simulink model "robo_arm_with_control"  (R2018b)
settings: Solver=VariableStepAuto  StartTime=0.0  StopTime=100  RelTol=1e-3  EnableMultiTasking=on
model workspace (MAT data in the model file):
  MCOS : class17 (value not decoded)
undefined symbols (not defined in the file): A_piston, base_rail_height, base_rail_lenth, base_rail_width, border_width_col, box_size_a, D, damp_mech, feedback_loop_gain, first_arm_height, first_arm_length, first_arm_mass, first_arm_width, gearbox_damping_factor, I, jaw_height, jaw_lenght, jaw_mass, jaw_width, K, L_piston, list_of_coordinates_x, list_of_coordinates_y, mechanical_hardstop_constraint, P, pinion_radius, rp_damping_factor, second_arm_height, second_arm_length, second_arm_mass, second_arm_width, third_arm_height, third_arm_length, third_arm_mass, third_arm_width, total_x, winding_resistance, X, x_init, x_max, Y, Z
libraries: fl_lib x47, sm_lib x34, nesl_utility x30, simulink x1, elec_lib x1, SimscapeFluids_lib x1
(part 3 of 3)

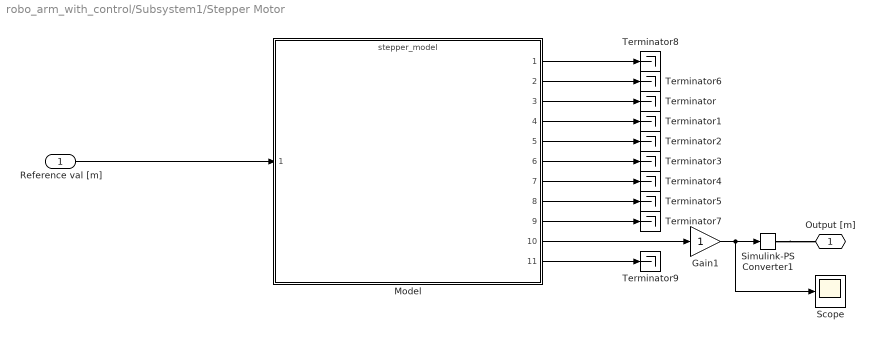
== system robo_arm_with_control/Subsystem1/Stepper Motor  ==
  Reference val [m] : Inport
  Gain1 : Gain
  Model : ModelReference  ModelNameDialog=stepper_model.slx  SimulationMode=Normal  ModelReferenceVersion=1.65
  Scope : Scope
  Simulink-PS Converter1 : nesl_utility/Simulink-PS Converter  PhysicalDomain=network_engine_domain  SubClassName=ps_input  LeftPortType=input  RightPortType=output  PseudoPeriodic=off  Frequencies=[]  NoiseDistribution=none  NoiseParameters=[]  Unit=m  AffineConversion=off  FilteringAndDerivatives=filter  SimscapeFilterOrder=2  InputFilterTimeConstant=0.001  UdotUserProvided=0
  Terminator{,1..9} (10 alike) : Terminator
  Output [m] : PMIOPort  Side=Right
  wires:
  Gain1/1 -> Scope/1, Simulink-PS Converter1/1
  Model/2 -> Terminator6/1
  Model/1 -> Terminator8/1
  Model/3 -> Terminator/1
  Model/4 -> Terminator1/1
  Model/7 -> Terminator4/1
  Model/8 -> Terminator5/1
  Model/9 -> Terminator7/1
  Model/6 -> Terminator3/1
  Model/5 -> Terminator2/1
  Model/11 -> Terminator9/1
  Model/10 -> Gain1/1
  Reference val [m]/1 -> Model/1
  connections:
  Simulink-PS Converter1/RConn1 -- Output [m]/RConn1

== system robo_arm_with_control/Subsystem1/UP//DOWN ==
  Prismatic Joint1 : sm_lib/Joints/Prismatic Joint  SenseConstraintForce=off  SenseConstraintForceX=off  SenseConstraintForceY=off  SenseConstraintForceZ=off  SenseConstraintTorque=off  SenseConstraintTorqueX=off  SenseConstraintTorqueY=off  SenseConstraintTorqueZ=off  SenseTotalForce=off  SenseTotalForceX=off  SenseTotalForceY=off  SenseTotalForceZ=off  SenseTotalTorque=off  SenseTotalTorqueX=off  SenseTotalTorqueY=off  SenseTotalTorqueZ=off  CompositeWrenchDir=FollowerOnBase  CompositeWrenchFrame=BaseFrame  EquilibriumPosition=0  EquilibriumPositionUnits=cm  SpringStiffness=0  SpringStiffnessUnits=N/m  DampingCoefficient=0  DampingCoefficientUnits=N/(m/s)  TorqueActuationMode=ComputedTorque  MotionActuationMode=InputMotion  SensePosition=on  SenseVelocity=off  SenseAcceleration=off  SenseTorqueForce=off  PositionTargetSpecify=off  PositionTargetPriority=High  PositionTargetValue=0  PositionTargetValueUnits=m  VelocityTargetSpecify=off  VelocityTargetPriority=High  VelocityTargetValue=0  VelocityTargetValueUnits=m/s
  In : PMIOPort  Side=Right
  Out : PMIOPort  Port=2  Side=Right
  Ang. Pos. In : PMIOPort  Port=3  Side=Right
  Pos_Out : PMIOPort  Port=4  Side=Right
  connections:
  Prismatic Joint1/LConn1 -- In/RConn1
  Prismatic Joint1/RConn1 -- Out/RConn1
  Ang. Pos. In/RConn1 -- Prismatic Joint1/LConn2
  Pos_Out/RConn1 -- Prismatic Joint1/RConn2

== system robo_arm_with_control/Subsystem1/X Servo ==
  Prismatic Joint : sm_lib/Joints/Prismatic Joint  SenseConstraintForce=off  SenseConstraintForceX=off  SenseConstraintForceY=off  SenseConstraintForceZ=off  SenseConstraintTorque=off  SenseConstraintTorqueX=off  SenseConstraintTorqueY=off  SenseConstraintTorqueZ=off  SenseTotalForce=off  SenseTotalForceX=off  SenseTotalForceY=off  SenseTotalForceZ=off  SenseTotalTorque=off  SenseTotalTorqueX=off  SenseTotalTorqueY=off  SenseTotalTorqueZ=off  CompositeWrenchDir=FollowerOnBase  CompositeWrenchFrame=BaseFrame  EquilibriumPosition=0  EquilibriumPositionUnits=cm  SpringStiffness=x_stiffness  SpringStiffnessUnits=N/m  DampingCoefficient=x_damping  DampingCoefficientUnits=N/(m/s)  TorqueActuationMode=ComputedTorque  MotionActuationMode=InputMotion  SensePosition=on  SenseVelocity=off  SenseAcceleration=off  SenseTorqueForce=off  PositionTargetSpecify=off  PositionTargetPriority=High  PositionTargetValue=0  PositionTargetValueUnits=m  VelocityTargetSpecify=off  VelocityTargetPriority=High  VelocityTargetValue=0  VelocityTargetValueUnits=m/s
  Rigid Transform : sm_lib/Frames and Transforms/Rigid Transform  TranslationMethod=None  TranslationStandardOffset=0  TranslationLengthUnit=m  TranslationStandardAxis=+Z  TranslationCartesianOffset=[0 0 0]  TranslationROffset=0  TranslationROffsetUnits=m  TranslationZOffset=0  TranslationZOffsetUnits=m  TranslationThetaOffset=0  TranslationThetaOffsetUnits=deg  RotationMethod=StandardAxis  RotationAngleUnits=deg  RotationStandardAxis=+Y  RotationAngle=90  RotationArbitraryAxis=[0 0 1]  FollAlignAxisA=+X  BaseAlignAxisA=+Y  FollAlignAxisB=+Y  BaseAlignAxisB=+Z  RotationSequenceAxes=FollowerAxes  RotationSequence=XYX  RotationSequenceAngles=[0 0 0]  RotationSequenceAnglesUnits=deg  RotationMatrix=[1 0 0; 0 1 0; 0 0 1]
  Rigid Transform1 : sm_lib/Frames and Transforms/Rigid Transform  TranslationMethod=None  TranslationStandardOffset=0  TranslationLengthUnit=m  TranslationStandardAxis=+Z  TranslationCartesianOffset=[0 0 0]  TranslationROffset=0  TranslationROffsetUnits=m  TranslationZOffset=0  TranslationZOffsetUnits=m  TranslationThetaOffset=0  TranslationThetaOffsetUnits=deg  RotationMethod=StandardAxis  RotationAngleUnits=deg  RotationStandardAxis=+Y  RotationAngle=90  RotationArbitraryAxis=[0 0 1]  FollAlignAxisA=+X  BaseAlignAxisA=+Y  FollAlignAxisB=+Y  BaseAlignAxisB=+Z  RotationSequenceAxes=FollowerAxes  RotationSequence=XYX  RotationSequenceAngles=[0 0 0]  RotationSequenceAnglesUnits=deg  RotationMatrix=[1 0 0; 0 1 0; 0 0 1]
  In : PMIOPort  Side=Right
  Out : PMIOPort  Port=2  Side=Right
  Ang. Pos. Input : PMIOPort  Port=3  Side=Left
  Pos_Out : PMIOPort  Port=4  Side=Right
  connections:
  In/RConn1 -- Rigid Transform1/RConn1
  Prismatic Joint/LConn1 -- Rigid Transform1/LConn1
  Out/RConn1 -- Rigid Transform/RConn1
  Prismatic Joint/RConn1 -- Rigid Transform/LConn1
  Ang. Pos. Input/RConn1 -- Prismatic Joint/LConn2
  Pos_Out/RConn1 -- Prismatic Joint/RConn2

== system robo_arm_with_control/Subsystem1/Y Servo ==
  Prismatic Joint1 : sm_lib/Joints/Prismatic Joint  SenseConstraintForce=off  SenseConstraintForceX=off  SenseConstraintForceY=off  SenseConstraintForceZ=off  SenseConstraintTorque=off  SenseConstraintTorqueX=off  SenseConstraintTorqueY=off  SenseConstraintTorqueZ=off  SenseTotalForce=off  SenseTotalForceX=off  SenseTotalForceY=off  SenseTotalForceZ=off  SenseTotalTorque=off  SenseTotalTorqueX=off  SenseTotalTorqueY=off  SenseTotalTorqueZ=off  CompositeWrenchDir=FollowerOnBase  CompositeWrenchFrame=BaseFrame  EquilibriumPosition=0  EquilibriumPositionUnits=cm  SpringStiffness=0  SpringStiffnessUnits=N/m  DampingCoefficient=0  DampingCoefficientUnits=N/(m/s)  TorqueActuationMode=ComputedTorque  MotionActuationMode=InputMotion  SensePosition=on  SenseVelocity=off  SenseAcceleration=off  SenseTorqueForce=off  PositionTargetSpecify=off  PositionTargetPriority=High  PositionTargetValue=0  PositionTargetValueUnits=m  VelocityTargetSpecify=off  VelocityTargetPriority=High  VelocityTargetValue=0  VelocityTargetValueUnits=m/s
  Rigid Transform3 : sm_lib/Frames and Transforms/Rigid Transform  TranslationMethod=None  TranslationStandardOffset=0  TranslationLengthUnit=m  TranslationStandardAxis=+Z  TranslationCartesianOffset=[0 0 0]  TranslationROffset=0  TranslationROffsetUnits=m  TranslationZOffset=0  TranslationZOffsetUnits=m  TranslationThetaOffset=0  TranslationThetaOffsetUnits=deg  RotationMethod=StandardAxis  RotationAngleUnits=deg  RotationStandardAxis=-X  RotationAngle=90  RotationArbitraryAxis=[0 0 1]  FollAlignAxisA=+X  BaseAlignAxisA=+Y  FollAlignAxisB=+Y  BaseAlignAxisB=+Z  RotationSequenceAxes=FollowerAxes  RotationSequence=XYX  RotationSequenceAngles=[0 0 0]  RotationSequenceAnglesUnits=deg  RotationMatrix=[1 0 0; 0 1 0; 0 0 1]
  Rigid Transform4 : sm_lib/Frames and Transforms/Rigid Transform  TranslationMethod=None  TranslationStandardOffset=0  TranslationLengthUnit=m  TranslationStandardAxis=+Z  TranslationCartesianOffset=[0 0 0]  TranslationROffset=0  TranslationROffsetUnits=m  TranslationZOffset=0  TranslationZOffsetUnits=m  TranslationThetaOffset=0  TranslationThetaOffsetUnits=deg  RotationMethod=StandardAxis  RotationAngleUnits=deg  RotationStandardAxis=-X  RotationAngle=90  RotationArbitraryAxis=[0 0 1]  FollAlignAxisA=+X  BaseAlignAxisA=+Y  FollAlignAxisB=+Y  BaseAlignAxisB=+Z  RotationSequenceAxes=FollowerAxes  RotationSequence=XYX  RotationSequenceAngles=[0 0 0]  RotationSequenceAnglesUnits=deg  RotationMatrix=[1 0 0; 0 1 0; 0 0 1]
  In : PMIOPort  Side=Right
  Out : PMIOPort  Port=2  Side=Right
  Ang. Pos. In : PMIOPort  Port=3  Side=Right
  Pos_Out : PMIOPort  Port=4  Side=Right
  connections:
  In/RConn1 -- Rigid Transform4/RConn1
  Prismatic Joint1/RConn1 -- Rigid Transform3/LConn1
  Prismatic Joint1/LConn1 -- Rigid Transform4/LConn1
  Out/RConn1 -- Rigid Transform3/RConn1
  Ang. Pos. In/RConn1 -- Prismatic Joint1/LConn2
  Prismatic Joint1/RConn2 -- Pos_Out/RConn1

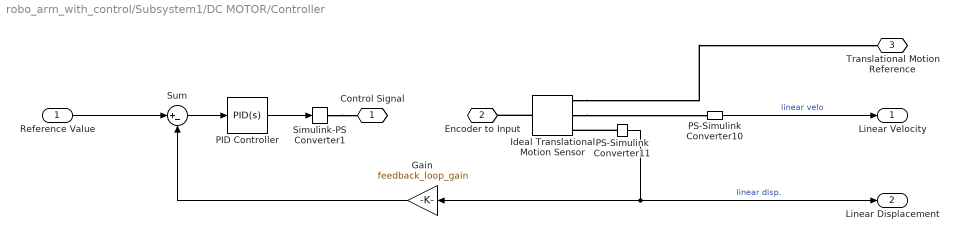
== system robo_arm_with_control/Subsystem1/DC MOTOR/Controller ==
  Reference Value : Inport
  Gain : Gain  Gain=feedback_loop_gain
  Ideal Translational Motion Sensor : fl_lib/Mechanical/Mechanical Sensors/Ideal Translational Motion Sensor  offset=0 m
  PID Controller : simulink/Continuous/PID Controller  Controller=PID  Form=Parallel  TimeDomain=Continuous-time  SampleTime=-1  IntegratorMethod=Forward Euler  FilterMethod=Forward Euler  ControllerParametersSource=internal  P=P  I=I  D=D  UseFilter=on  N=100  TunerSelectOption=Transfer Function Based (PID Tuner App)  InitialConditionSource=internal  InitialConditionForIntegrator=0  InitialConditionForFilter=0  DifferentiatorICPrevScaledInput=0  ExternalReset=none  TrackingMode=off  Kt=1  LimitOutput=off  UpperSaturationLimit=inf  LowerSaturationLimit=-inf  LinearizeAsGain=on  AntiWindupMode=none  Kb=1  POutMin=[]  POutMax=[]  IOutMin=[]  IOutMax=[]  DOutMin=[]  DOutMax=[]  NOutMin=[]  NOutMax=[]  SumOutMin=[]  SumOutMax=[]  SaturationOutMin=[]  SaturationOutMax=[]  PParamMin=[]  PParamMax=[]  IParamMin=[]  IParamMax=[]  DParamMin=[]  DParamMax=[]  NParamMin=[]  NParamMax=[]  KbParamMin=[]  KbParamMax=[]  KtParamMin=[]  KtParamMax=[]  KbOutMin=[]  KbOutMax=[]  KtOutMin=[]  KtOutMax=[]  IntegratorOutMin=[]  IntegratorOutMax=[]  FilterOutMin=[]  FilterOutMax=[]  SumI1OutMin=[]  SumI1OutMax=[]  SumI2OutMin=[]  SumI2OutMax=[]  SumI3OutMin=[]  SumI3OutMax=[]  SumI4OutMin=[]  SumI4OutMax=[]  SumDOutMin=[]  SumDOutMax=[]  DifferentiatorOutMin=[]  DifferentiatorOutMax=[]  FilterDiffOutCoefMin=[]  FilterDiffOutCoefMax=[]  ReciprocalOutMin=[]  ReciprocalOutMax=[]  SumDenOutMin=[]  SumDenOutMax=[]  SumNumOutMin=[]  SumNumOutMax=[]  DivideOutMin=[]  DivideOutMax=[]  IntegratorContinuousStateAttributes=''  IntegratorStateMustResolveToSignalObject=off  IntegratorRTWStateStorageClass=Auto  FilterContinuousStateAttributes=''  FilterStateMustResolveToSignalObject=off  FilterRTWStateStorageClass=Auto  ParallelPVariant=InternalParameters  IdealPVariant=Disabled  IVariant=InternalParameters  DVariant=InternalParameters  IntegratorVariant=Continuous  SatVariant=Disabled  AWVariant=Passthrough  PCopyVariant=Disabled  TRVariant=Disabled  FdbkBlocksVariant=Forward  IdealPFdbkVariant=Disabled  SatFdbkVariant=Disabled  DerivativeFilterVariant=ContFilter  NVariant=InternalParameters  NCopyVariant=Disabled  FilterICVariant=InternalICsFilter  IntegratorICVariant=InternalICs  ExternalResetVariant=Disabled  TRSumVariant=Passthrough  SumFdbkVariant=Disabled  SumVariant=Sum_PID
  PS-Simulink Converter10 : nesl_utility/PS-Simulink Converter  PhysicalDomain=network_engine_domain  SubClassName=ps_output  LeftPortType=input  RightPortType=output  PseudoPeriodic=off  Frequencies=[]  Unit=1  AffineConversion=off
  PS-Simulink Converter11 : nesl_utility/PS-Simulink Converter  PhysicalDomain=network_engine_domain  SubClassName=ps_output  LeftPortType=input  RightPortType=output  PseudoPeriodic=off  Frequencies=[]  Unit=m  AffineConversion=off
  Simulink-PS Converter1 : nesl_utility/Simulink-PS Converter  PhysicalDomain=network_engine_domain  SubClassName=ps_input  LeftPortType=input  RightPortType=output  PseudoPeriodic=off  Frequencies=[]  NoiseDistribution=none  NoiseParameters=[]  Unit=1  AffineConversion=off  FilteringAndDerivatives=filter  SimscapeFilterOrder=1  InputFilterTimeConstant=0.001  UdotUserProvided=0
  Sum : Sum  Inputs=|+-
  Control Signal : PMIOPort  Side=Right
  Encoder to Input : PMIOPort  Port=2  Side=Left
  Translational Motion Reference : PMIOPort  Port=3  Side=Left
  Linear Velocity : Outport
  Linear Displacement : Outport  Port=2
  wires:
  Reference Value/1 -> Sum/1
  PS-Simulink Converter11/1 -> Linear Displacement/1, Gain/1  "linear disp."
  PID Controller/1 -> Simulink-PS Converter1/1
  Sum/1 -> PID Controller/1
  Gain/1 -> Sum/2
  PS-Simulink Converter10/1 -> Linear Velocity/1  "linear velo"
  connections:
  Ideal Translational Motion Sensor/RConn1 -- Translational Motion Reference/RConn1
  Simulink-PS Converter1/RConn1 -- Control Signal/RConn1
  PS-Simulink Converter11/LConn1 -- Ideal Translational Motion Sensor/RConn3
  Ideal Translational Motion Sensor/LConn1 -- Encoder to Input/RConn1
  Ideal Translational Motion Sensor/RConn2 -- PS-Simulink Converter10/LConn1

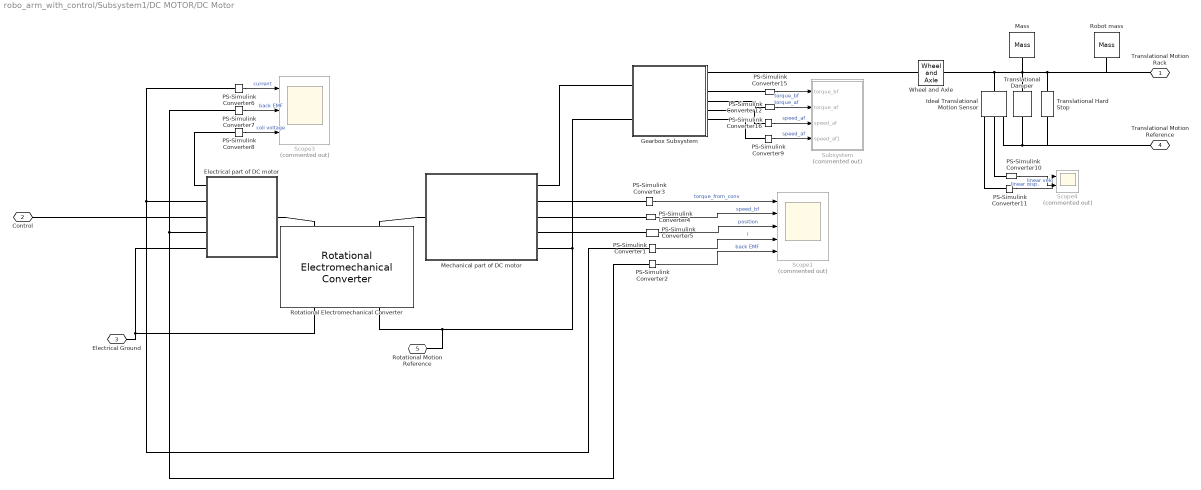
== system robo_arm_with_control/Subsystem1/DC MOTOR/DC Motor ==
  Electrical part of DC motor : Subsystem
  Gearbox Subsystem : Subsystem
  Ideal Translational Motion Sensor : fl_lib/Mechanical/Mechanical Sensors/Ideal Translational Motion Sensor  offset=0 m
  Mass : fl_lib/Mechanical/Translational Elements/Mass  mass=rack_mass kg  v_specify=off  v_priority=High  v=0 m/s  v_nominal_specify=off  v_nominal_unit=m/s  v_nominal_value=1  f_specify=off  f_priority=None  f=0 N  f_nominal_specify=off  f_nominal_unit=N  f_nominal_value=1
  Mechanical part of DC motor : Subsystem
  PS-Simulink Converter{1..12,15..16} (14 alike) : nesl_utility/PS-Simulink Converter  PhysicalDomain=network_engine_domain  SubClassName=ps_output  LeftPortType=input  RightPortType=output  PseudoPeriodic=off  Frequencies=[]  Unit=1  AffineConversion=off
  Robot mass : fl_lib/Mechanical/Translational Elements/Mass  mass=first_arm_mass + second_arm_mass + third_arm_mass + jaw_mass*2 kg  v_specify=off  v_priority=High  v=0 m/s  v_nominal_specify=off  v_nominal_unit=m/s  v_nominal_value=1  f_specify=off  f_priority=None  f=0 N  f_nominal_specify=off  f_nominal_unit=N  f_nominal_value=1
  Rotational Electromechanical Converter : fl_lib/Electrical/Electrical Elements/Rotational Electromechanical Converter  K=K V/rpm  i_specify=off  i_priority=None  i=0 A  i_nominal_specify=off  i_nominal_unit=A  i_nominal_value=1  v_specify=off  v_priority=None  v=0 V  v_nominal_specify=off  v_nominal_unit=V  v_nominal_value=1  t_specify=off  t_priority=None  t=0 N*m  t_nominal_specify=off  t_nominal_unit=N*m  t_nominal_value=1  w_specify=off  w_priority=None  w=0 rad/s  w_nominal_specify=off  w_nominal_unit=rad/s  w_nominal_value=1
      settings: SourceProductName=Simscape
  Scope1 : Scope  Commented=on  NumInputPorts=5
  Scope3 : Scope  Commented=on  NumInputPorts=3
  Scope4 : Scope  Commented=on  NumInputPorts=2
  Subsystem : Subsystem  Commented=on
  Translational Damper : fl_lib/Mechanical/Translational Elements/Translational Damper  D=rp_damping_factor N/(m/s)  v_specify=off  v_priority=None  v=0 m/s  v_nominal_specify=off  v_nominal_unit=m/s  v_nominal_value=1  f_specify=off  f_priority=None  f=0 N  f_nominal_specify=off  f_nominal_unit=N  f_nominal_value=1
  Translational Hard Stop : fl_lib/Mechanical/Translational Elements/Translational Hard Stop  upper_bnd=mechanical_hardstop_constraint m  lower_bnd=-mechanical_hardstop_constraint m  stiff_up=1e6 N/m  stiff_low=1e6 N/m  D_up=150 N/(m/s)  D_low=150 N/(m/s)  model=1  transition=0.1 mm  v_specify=off  v_priority=None  v=0 m/s  v_nominal_specify=off  v_nominal_unit=m/s  v_nominal_value=1  f_specify=off  f_priority=None  f=0 N  f_nominal_specify=off  f_nominal_unit=N  f_nominal_value=1  x_specify=off  x_priority=High  x=0 m  x_nominal_specify=off  x_nominal_unit=m  x_nominal_value=1
  Wheel and Axle : fl_lib/Mechanical/Mechanisms/Wheel and Axle  R=pinion_radius m  or=1  t_specify=off  t_priority=None  t=0 N*m  t_nominal_specify=off  t_nominal_unit=N*m  t_nominal_value=1  f_specify=off  f_priority=None  f=0 N  f_nominal_specify=off  f_nominal_unit=N  f_nominal_value=1
      settings: SourceProductName=Simscape
  Translational Motion Rack : PMIOPort  Side=Right
  Control : PMIOPort  Port=2  Side=Left
  Electrical Ground : PMIOPort  Port=3  Side=Left
  Translational Motion Reference : PMIOPort  Port=4  Side=Left
  Rotational Motion Reference : PMIOPort  Port=5  Side=Left
  wires:
  PS-Simulink Converter1/1 -> Scope1/4  "i"
  PS-Simulink Converter8/1 -> Scope3/3  "coil voltage"
  PS-Simulink Converter15/1 -> Subsystem/1(torque_bf)  "torque_bf"
  PS-Simulink Converter5/1 -> Scope1/3  "position"
  PS-Simulink Converter6/1 -> Scope3/1  "current"
  PS-Simulink Converter9/1 -> Subsystem/4(speed_af1)  "speed_af"
  PS-Simulink Converter7/1 -> Scope3/2  "back EMF"
  PS-Simulink Converter3/1 -> Scope1/1  "torque_from_conv"
  PS-Simulink Converter2/1 -> Scope1/5  "back EMF"
  PS-Simulink Converter11/1 -> Scope4/1  "linear disp."
  PS-Simulink Converter16/1 -> Subsystem/3(speed_af)  "speed_af"
  PS-Simulink Converter10/1 -> Scope4/2  "linear velo"
  PS-Simulink Converter12/1 -> Subsystem/2(torque_af)  "torque_af"
  PS-Simulink Converter4/1 -> Scope1/2  "speed_bf"
  connections:
  Gearbox Subsystem/RConn4 -- PS-Simulink Converter12/LConn1
  Rotational Electromechanical Converter/RConn1 -- Electrical part of DC motor/RConn5 -- Electrical Ground/RConn1
  PS-Simulink Converter4/LConn1 -- Mechanical part of DC motor/RConn3
  PS-Simulink Converter9/LConn1 -- Gearbox Subsystem/RConn6
  Ideal Translational Motion Sensor/RConn3 -- PS-Simulink Converter11/LConn1
  Control/RConn1 -- Electrical part of DC motor/RConn3
  PS-Simulink Converter5/LConn1 -- Mechanical part of DC motor/RConn4
  PS-Simulink Converter16/LConn1 -- Gearbox Subsystem/RConn5
  PS-Simulink Converter6/LConn1 -- PS-Simulink Converter1/LConn1 -- Electrical part of DC motor/RConn2
  Ideal Translational Motion Sensor/LConn1 -- Translational Motion Rack/RConn1 -- Robot mass/LConn1 -- Translational Hard Stop/LConn1 -- Mass/LConn1 -- Translational Damper/LConn1 -- Wheel and Axle/RConn1
  Electrical part of DC motor/LConn1 -- Rotational Electromechanical Converter/LConn1
  PS-Simulink Converter7/LConn1 -- Electrical part of DC motor/RConn4 -- PS-Simulink Converter2/LConn1
  Mechanical part of DC motor/LConn1 -- Rotational Electromechanical Converter/LConn2
  Gearbox Subsystem/LConn1 -- Mechanical part of DC motor/RConn1
  PS-Simulink Converter15/LConn1 -- Gearbox Subsystem/RConn3
  Translational Damper/RConn1 -- Translational Motion Reference/RConn1 -- Translational Hard Stop/RConn1 -- Ideal Translational Motion Sensor/RConn1
  Gearbox Subsystem/LConn2 -- Mechanical part of DC motor/RConn5 -- Rotational Motion Reference/RConn1 -- Rotational Electromechanical Converter/RConn2
  Ideal Translational Motion Sensor/RConn2 -- PS-Simulink Converter10/LConn1
  Mechanical part of DC motor/RConn2 -- PS-Simulink Converter3/LConn1
  Wheel and Axle/LConn1 -- Gearbox Subsystem/RConn1
  Electrical part of DC motor/RConn1 -- PS-Simulink Converter8/LConn1

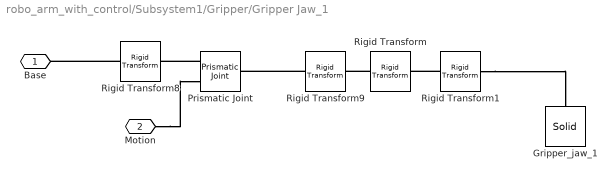
== system robo_arm_with_control/Subsystem1/Gripper/Gripper Jaw_1 ==
  Gripper_jaw_1 : sm_lib/Body Elements/Solid  InertiaType=CalculateFromGeometry  Mass=1  MassUnits=kg  CenterOfMass=[0 0 0]  CenterOfMassUnits=m  MomentsOfInertia=[1 1 1]  MomentsOfInertiaUnits=kg*m^2  ProductsOfInertia=[0 0 0]  ProductsOfInertiaUnits=kg*m^2  BasedOnType=Density  Density=jaw_density  DensityUnits=kg/m^3  DoExposeReferenceFrame=on  SerializedFrames=<Frames/>  GraphicType=FromGeometry  MarkerShape=Sphere  MarkerSize=10  GraphicVisPropType=SimpleVisualProperties  GraphicDiffuseColor=[0.5 0.5 0.5]  GraphicSpecularColor=[0.5 0.5 0.5 1.0]  GraphicAmbientColor=[0.15 0.15 0.15 1.0]  GraphicEmissiveColor=[0.0 0.0 0.0 1.0]  GraphicShininess=75  GraphicOpacity=1.0  GeometryShape=Brick  RectangleSize=[1 1]  RectangleSizeUnits=m  BrickDimensions=[jaw_width jaw_lenght jaw_height]  BrickDimensionUnits=cm  CylinderRadius=1  CylinderRadiusUnits=m  CylinderLength=1  CylinderLengthUnits=m  SphereRadius=1  SphereRadiusUnits=m  EllipsoidRadii=[1 1 1]  EllipsoidRadiiUnits=m  ExtrusionCrossSection=[1 1; -1 1; -1 -1; 1 -1]  ExtrusionCrossSectionUnits=m  ExtrusionLength=1  ExtrusionLengthUnits=m  PolygonNumSides=3  PolygonOuterRadius=1  PolygonOuterRadiusUnits=m  ExtGeomFileType=STEP  ExtGeomFileUnits=m  RevolutionCrossSection=[1 1; 1 -1; 2 -1; 2 1]  RevolutionCrossSectionUnits=m  RevolutionExtent=Full  RevolutionAngle=180  RevolutionAngleUnits=deg
  Prismatic Joint : sm_lib/Joints/Prismatic Joint  SenseConstraintForce=off  SenseConstraintForceX=off  SenseConstraintForceY=off  SenseConstraintForceZ=off  SenseConstraintTorque=off  SenseConstraintTorqueX=off  SenseConstraintTorqueY=off  SenseConstraintTorqueZ=off  SenseTotalForce=off  SenseTotalForceX=off  SenseTotalForceY=off  SenseTotalForceZ=off  SenseTotalTorque=off  SenseTotalTorqueX=off  SenseTotalTorqueY=off  SenseTotalTorqueZ=off  CompositeWrenchDir=FollowerOnBase  CompositeWrenchFrame=BaseFrame  EquilibriumPosition=0  EquilibriumPositionUnits=m  SpringStiffness=0  SpringStiffnessUnits=N/m  DampingCoefficient=0  DampingCoefficientUnits=N/(m/s)  TorqueActuationMode=ComputedTorque  MotionActuationMode=InputMotion  SensePosition=off  SenseVelocity=off  SenseAcceleration=off  SenseTorqueForce=off  PositionTargetSpecify=off  PositionTargetPriority=High  PositionTargetValue=0  PositionTargetValueUnits=m  VelocityTargetSpecify=off  VelocityTargetPriority=High  VelocityTargetValue=0  VelocityTargetValueUnits=m/s
  Rigid Transform : sm_lib/Frames and Transforms/Rigid Transform  TranslationMethod=StandardAxis  TranslationStandardOffset=third_arm_height/2+jaw_height/2  TranslationLengthUnit=cm  TranslationStandardAxis=+Z  TranslationCartesianOffset=[0 0 0]  TranslationROffset=0  TranslationROffsetUnits=m  TranslationZOffset=0  TranslationZOffsetUnits=m  TranslationThetaOffset=0  TranslationThetaOffsetUnits=deg  RotationMethod=None  RotationAngleUnits=deg  RotationStandardAxis=-Z  RotationAngle=0.0  RotationArbitraryAxis=[0 0 1]  FollAlignAxisA=+X  BaseAlignAxisA=+Y  FollAlignAxisB=+Y  BaseAlignAxisB=+Z  RotationSequenceAxes=FollowerAxes  RotationSequence=XYX  RotationSequenceAngles=[0 0 0]  RotationSequenceAnglesUnits=deg  RotationMatrix=[1 0 0; 0 1 0; 0 0 1]
  Rigid Transform1 : sm_lib/Frames and Transforms/Rigid Transform  TranslationMethod=StandardAxis  TranslationStandardOffset=third_arm_length/2+jaw_width/2  TranslationLengthUnit=cm  TranslationStandardAxis=+X  TranslationCartesianOffset=[0 0 0]  TranslationROffset=0  TranslationROffsetUnits=m  TranslationZOffset=0  TranslationZOffsetUnits=m  TranslationThetaOffset=0  TranslationThetaOffsetUnits=deg  RotationMethod=None  RotationAngleUnits=deg  RotationStandardAxis=+Z  RotationAngle=0.0  RotationArbitraryAxis=[0 0 1]  FollAlignAxisA=+X  BaseAlignAxisA=+Y  FollAlignAxisB=+Y  BaseAlignAxisB=+Z  RotationSequenceAxes=FollowerAxes  RotationSequence=XYX  RotationSequenceAngles=[0 0 0]  RotationSequenceAnglesUnits=deg  RotationMatrix=[1 0 0; 0 1 0; 0 0 1]
  Rigid Transform8 : sm_lib/Frames and Transforms/Rigid Transform  TranslationMethod=None  TranslationStandardOffset=0  TranslationLengthUnit=m  TranslationStandardAxis=+Z  TranslationCartesianOffset=[0 0 0]  TranslationROffset=0  TranslationROffsetUnits=m  TranslationZOffset=0  TranslationZOffsetUnits=m  TranslationThetaOffset=0  TranslationThetaOffsetUnits=deg  RotationMethod=StandardAxis  RotationAngleUnits=deg  RotationStandardAxis=+Y  RotationAngle=90  RotationArbitraryAxis=[0 0 1]  FollAlignAxisA=+X  BaseAlignAxisA=+Y  FollAlignAxisB=+Y  BaseAlignAxisB=+Z  RotationSequenceAxes=FollowerAxes  RotationSequence=XYX  RotationSequenceAngles=[0 0 0]  RotationSequenceAnglesUnits=deg  RotationMatrix=[1 0 0; 0 1 0; 0 0 1]
  Rigid Transform9 : sm_lib/Frames and Transforms/Rigid Transform  TranslationMethod=None  TranslationStandardOffset=0  TranslationLengthUnit=m  TranslationStandardAxis=+Z  TranslationCartesianOffset=[0 0 0]  TranslationROffset=0  TranslationROffsetUnits=m  TranslationZOffset=0  TranslationZOffsetUnits=m  TranslationThetaOffset=0  TranslationThetaOffsetUnits=deg  RotationMethod=StandardAxis  RotationAngleUnits=deg  RotationStandardAxis=+Y  RotationAngle=90  RotationArbitraryAxis=[0 0 1]  FollAlignAxisA=+X  BaseAlignAxisA=+Y  FollAlignAxisB=+Y  BaseAlignAxisB=+Z  RotationSequenceAxes=FollowerAxes  RotationSequence=XYX  RotationSequenceAngles=[0 0 0]  RotationSequenceAnglesUnits=deg  RotationMatrix=[1 0 0; 0 1 0; 0 0 1]
  Base : PMIOPort  Side=Left
  Motion : PMIOPort  Port=2  Side=Left
  connections:
  Rigid Transform/LConn1 -- Rigid Transform9/LConn1
  Rigid Transform1/LConn1 -- Rigid Transform/RConn1
  Rigid Transform8/LConn1 -- Base/RConn1
  Rigid Transform1/RConn1 -- Gripper_jaw_1/RConn1
  Prismatic Joint/LConn1 -- Rigid Transform8/RConn1
  Rigid Transform9/RConn1 -- Prismatic Joint/RConn1
  Motion/RConn1 -- Prismatic Joint/LConn2

== system robo_arm_with_control/Subsystem1/Gripper/Gripper Jaw_2 ==
  Gripper_jaw_2 : sm_lib/Body Elements/Solid  InertiaType=CalculateFromGeometry  Mass=1  MassUnits=kg  CenterOfMass=[0 0 0]  CenterOfMassUnits=m  MomentsOfInertia=[1 1 1]  MomentsOfInertiaUnits=kg*m^2  ProductsOfInertia=[0 0 0]  ProductsOfInertiaUnits=kg*m^2  BasedOnType=Density  Density=jaw_density  DensityUnits=kg/m^3  DoExposeReferenceFrame=on  SerializedFrames=<Frames/>  GraphicType=FromGeometry  MarkerShape=Sphere  MarkerSize=10  GraphicVisPropType=SimpleVisualProperties  GraphicDiffuseColor=[0.5 0.5 0.5]  GraphicSpecularColor=[0.5 0.5 0.5 1.0]  GraphicAmbientColor=[0.15 0.15 0.15 1.0]  GraphicEmissiveColor=[0.0 0.0 0.0 1.0]  GraphicShininess=75  GraphicOpacity=1.0  GeometryShape=Brick  RectangleSize=[1 1]  RectangleSizeUnits=m  BrickDimensions=[jaw_width jaw_lenght jaw_height]  BrickDimensionUnits=cm  CylinderRadius=1  CylinderRadiusUnits=m  CylinderLength=1  CylinderLengthUnits=m  SphereRadius=1  SphereRadiusUnits=m  EllipsoidRadii=[1 1 1]  EllipsoidRadiiUnits=m  ExtrusionCrossSection=[1 1; -1 1; -1 -1; 1 -1]  ExtrusionCrossSectionUnits=m  ExtrusionLength=1  ExtrusionLengthUnits=m  PolygonNumSides=3  PolygonOuterRadius=1  PolygonOuterRadiusUnits=m  ExtGeomFileType=STEP  ExtGeomFileUnits=m  RevolutionCrossSection=[1 1; 1 -1; 2 -1; 2 1]  RevolutionCrossSectionUnits=m  RevolutionExtent=Full  RevolutionAngle=180  RevolutionAngleUnits=deg
  Prismatic Joint1 : sm_lib/Joints/Prismatic Joint  SenseConstraintForce=off  SenseConstraintForceX=off  SenseConstraintForceY=off  SenseConstraintForceZ=off  SenseConstraintTorque=off  SenseConstraintTorqueX=off  SenseConstraintTorqueY=off  SenseConstraintTorqueZ=off  SenseTotalForce=off  SenseTotalForceX=off  SenseTotalForceY=off  SenseTotalForceZ=off  SenseTotalTorque=off  SenseTotalTorqueX=off  SenseTotalTorqueY=off  SenseTotalTorqueZ=off  CompositeWrenchDir=FollowerOnBase  CompositeWrenchFrame=BaseFrame  EquilibriumPosition=0  EquilibriumPositionUnits=m  SpringStiffness=0  SpringStiffnessUnits=N/m  DampingCoefficient=0  DampingCoefficientUnits=N/(m/s)  TorqueActuationMode=ComputedTorque  MotionActuationMode=InputMotion  SensePosition=off  SenseVelocity=off  SenseAcceleration=off  SenseTorqueForce=off  PositionTargetSpecify=off  PositionTargetPriority=High  PositionTargetValue=0  PositionTargetValueUnits=m  VelocityTargetSpecify=off  VelocityTargetPriority=High  VelocityTargetValue=0  VelocityTargetValueUnits=m/s
  Rigid Transform10 : sm_lib/Frames and Transforms/Rigid Transform  TranslationMethod=None  TranslationStandardOffset=0  TranslationLengthUnit=m  TranslationStandardAxis=+Z  TranslationCartesianOffset=[0 0 0]  TranslationROffset=0  TranslationROffsetUnits=m  TranslationZOffset=0  TranslationZOffsetUnits=m  TranslationThetaOffset=0  TranslationThetaOffsetUnits=deg  RotationMethod=StandardAxis  RotationAngleUnits=deg  RotationStandardAxis=+Y  RotationAngle=90  RotationArbitraryAxis=[0 0 1]  FollAlignAxisA=+X  BaseAlignAxisA=+Y  FollAlignAxisB=+Y  BaseAlignAxisB=+Z  RotationSequenceAxes=FollowerAxes  RotationSequence=XYX  RotationSequenceAngles=[0 0 0]  RotationSequenceAnglesUnits=deg  RotationMatrix=[1 0 0; 0 1 0; 0 0 1]
  Rigid Transform11 : sm_lib/Frames and Transforms/Rigid Transform  TranslationMethod=None  TranslationStandardOffset=0  TranslationLengthUnit=m  TranslationStandardAxis=+Z  TranslationCartesianOffset=[0 0 0]  TranslationROffset=0  TranslationROffsetUnits=m  TranslationZOffset=0  TranslationZOffsetUnits=m  TranslationThetaOffset=0  TranslationThetaOffsetUnits=deg  RotationMethod=StandardAxis  RotationAngleUnits=deg  RotationStandardAxis=+Y  RotationAngle=90  RotationArbitraryAxis=[0 0 1]  FollAlignAxisA=+X  BaseAlignAxisA=+Y  FollAlignAxisB=+Y  BaseAlignAxisB=+Z  RotationSequenceAxes=FollowerAxes  RotationSequence=XYX  RotationSequenceAngles=[0 0 0]  RotationSequenceAnglesUnits=deg  RotationMatrix=[1 0 0; 0 1 0; 0 0 1]
  Rigid Transform3 : sm_lib/Frames and Transforms/Rigid Transform  TranslationMethod=StandardAxis  TranslationStandardOffset=third_arm_height/2+jaw_height/2  TranslationLengthUnit=cm  TranslationStandardAxis=+Z  TranslationCartesianOffset=[0 0 0]  TranslationROffset=0  TranslationROffsetUnits=m  TranslationZOffset=0  TranslationZOffsetUnits=m  TranslationThetaOffset=0  TranslationThetaOffsetUnits=deg  RotationMethod=None  RotationAngleUnits=deg  RotationStandardAxis=-Z  RotationAngle=0.0  RotationArbitraryAxis=[0 0 1]  FollAlignAxisA=+X  BaseAlignAxisA=+Y  FollAlignAxisB=+Y  BaseAlignAxisB=+Z  RotationSequenceAxes=FollowerAxes  RotationSequence=XYX  RotationSequenceAngles=[0 0 0]  RotationSequenceAnglesUnits=deg  RotationMatrix=[1 0 0; 0 1 0; 0 0 1]
  Rigid Transform4 : sm_lib/Frames and Transforms/Rigid Transform  TranslationMethod=StandardAxis  TranslationStandardOffset=-(jaw_width+jaw_width/2)  TranslationLengthUnit=cm  TranslationStandardAxis=+X  TranslationCartesianOffset=[0 0 0]  TranslationROffset=0  TranslationROffsetUnits=m  TranslationZOffset=0  TranslationZOffsetUnits=m  TranslationThetaOffset=0  TranslationThetaOffsetUnits=deg  RotationMethod=None  RotationAngleUnits=deg  RotationStandardAxis=+Z  RotationAngle=0.0  RotationArbitraryAxis=[0 0 1]  FollAlignAxisA=+X  BaseAlignAxisA=+Y  FollAlignAxisB=+Y  BaseAlignAxisB=+Z  RotationSequenceAxes=FollowerAxes  RotationSequence=XYX  RotationSequenceAngles=[0 0 0]  RotationSequenceAnglesUnits=deg  RotationMatrix=[1 0 0; 0 1 0; 0 0 1]
  B : PMIOPort  Side=Left
  Motion : PMIOPort  Port=2  Side=Left
  connections:
  Prismatic Joint1/LConn1 -- Rigid Transform10/RConn1
  Rigid Transform3/LConn1 -- Rigid Transform11/LConn1
  Prismatic Joint1/RConn1 -- Rigid Transform11/RConn1
  Motion/RConn1 -- Prismatic Joint1/LConn2
  Gripper_jaw_2/RConn1 -- Rigid Transform4/RConn1
  Rigid Transform4/LConn1 -- Rigid Transform3/RConn1
  Rigid Transform10/LConn1 -- B/RConn1

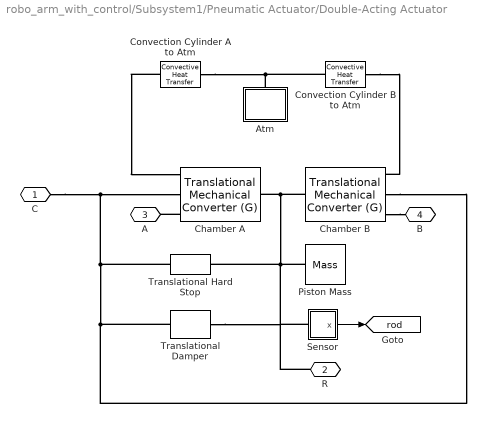
== system robo_arm_with_control/Subsystem1/Pneumatic Actuator/Double-Acting Actuator ==
  Atm : Subsystem
      mask Display: disp('Atm')
  Chamber A : fl_lib/Gas/Elements/Translational Mechanical Converter (G)  mech_orientation=1  interface_area=A_piston m^2  length_init=x_init m  dead_volume=0.1 * A_piston * x_max m^3  area_A=A_port m^2  environment_spec=1  environment_pressure=0.101325 MPa  p_converter_specify=on  p_converter_priority=High  p_converter=p_init MPa  p_converter_nominal_specify=off  p_converter_nominal_unit=MPa  p_converter_nominal_value=1  T_converter_specify=on  T_converter_priority=High  T_converter=T_init K  T_converter_nominal_specify=off  T_converter_nominal_unit=K  T_converter_nominal_value=1  rho_converter_specify=off  rho_converter_priority=None  rho_converter=1.2 kg/m^3  rho_converter_nominal_specify=off  rho_converter_nominal_unit=kg/m^3  rho_converter_nominal_value=1
      settings: SourceProductName=Simscape  SourceProductBaseCode=SS
  Chamber B : fl_lib/Gas/Elements/Translational Mechanical Converter (G)  mech_orientation=-1  interface_area=A_piston m^2  length_init=- x_max + x_init m  dead_volume=0.1 * A_piston * x_max m^3  area_A=A_port m^2  environment_spec=1  environment_pressure=0.101325 MPa  p_converter_specify=on  p_converter_priority=High  p_converter=p_init MPa  p_converter_nominal_specify=off  p_converter_nominal_unit=MPa  p_converter_nominal_value=1  T_converter_specify=on  T_converter_priority=High  T_converter=T_init K  T_converter_nominal_specify=off  T_converter_nominal_unit=K  T_converter_nominal_value=1  rho_converter_specify=off  rho_converter_priority=None  rho_converter=1.2 kg/m^3  rho_converter_nominal_specify=off  rho_converter_nominal_unit=kg/m^3  rho_converter_nominal_value=1
      settings: SourceProductName=Simscape  SourceProductBaseCode=SS
  Convection Cylinder A to Atm : fl_lib/Thermal/Thermal Elements/Convective Heat Transfer  area=2*A_piston + sqrt(pi*A_piston)*L_piston m^2  heat_tr_coeff=20 W/(m^2 * K)  T_specify=off  T_priority=None  T=0 K  T_nominal_specify=off  T_nominal_unit=K  T_nominal_value=1  Q_specify=off  Q_priority=None  Q=0 W  Q_nominal_specify=off  Q_nominal_unit=W  Q_nominal_value=1
  Convection Cylinder B to Atm : fl_lib/Thermal/Thermal Elements/Convective Heat Transfer  area=2*A_piston + sqrt(pi*A_piston)*L_piston m^2  heat_tr_coeff=20 W/(m^2 * K)  T_specify=off  T_priority=None  T=0 K  T_nominal_specify=off  T_nominal_unit=K  T_nominal_value=1  Q_specify=off  Q_priority=None  Q=0 W  Q_nominal_specify=off  Q_nominal_unit=W  Q_nominal_value=1
  Piston Mass : fl_lib/Mechanical/Translational Elements/Mass  mass=M_piston kg  v_specify=off  v_priority=High  v=0 m/s  v_nominal_specify=off  v_nominal_unit=m/s  v_nominal_value=1  f_specify=off  f_priority=None  f=0 N  f_nominal_specify=off  f_nominal_unit=N  f_nominal_value=1
  Sensor : Subsystem
      mask Display: disp('S')
  Translational Damper : fl_lib/Mechanical/Translational Elements/Translational Damper  D=damp_mech N/(m/s)  v_specify=off  v_priority=None  v=0 m/s  v_nominal_specify=off  v_nominal_unit=m/s  v_nominal_value=1  f_specify=off  f_priority=None  f=0 N  f_nominal_specify=off  f_nominal_unit=N  f_nominal_value=1
  Translational Hard Stop : fl_lib/Mechanical/Translational Elements/Translational Hard Stop  upper_bnd=x_max m  lower_bnd=0 m  stiff_up=stiff_hard_stop N/m  stiff_low=stiff_hard_stop N/m  D_up=damp_hard_stop N/(m/s)  D_low=damp_hard_stop N/(m/s)  model=3  transition=0.1 mm  v_specify=off  v_priority=None  v=0 m/s  v_nominal_specify=off  v_nominal_unit=m/s  v_nominal_value=1  f_specify=off  f_priority=None  f=0 N  f_nominal_specify=off  f_nominal_unit=N  f_nominal_value=1  x_specify=on  x_priority=High  x=x_init m  x_nominal_specify=off  x_nominal_unit=m  x_nominal_value=1
  C : PMIOPort  Side=Left
  R : PMIOPort  Port=2  Side=Right
  A : PMIOPort  Port=3  Side=Left
  B : PMIOPort  Port=4  Side=Right
  tag scope: rod=global
  wires:
  Sensor/1(x) -> [rod]
  connections:
  Chamber B/RConn1 -- R/RConn1 -- Sensor/LConn1 -- Translational Damper/LConn1 -- Piston Mass/LConn1 -- Translational Hard Stop/LConn1 -- Chamber A/RConn1
  Translational Hard Stop/RConn1 -- Chamber B/LConn2 -- Translational Damper/RConn1 -- C/RConn1 -- Chamber A/LConn2
  Chamber A/LConn1 -- A/RConn1
  Chamber B/LConn1 -- B/RConn1
  Convection Cylinder A to Atm/RConn1 -- Atm/RConn1 -- Convection Cylinder B to Atm/RConn1
  Convection Cylinder B to Atm/LConn1 -- Chamber B/LConn3
  Convection Cylinder A to Atm/LConn1 -- Chamber A/LConn3

== system robo_arm_with_control/Subsystem1/Pneumatic Actuator/Load ==
  Ideal Force Source : fl_lib/Mechanical/Mechanical Sources/Ideal Force Source
  Load Force : fl_lib/Physical Signals/Sources/PS Constant  constant=-500
  Mechanical Translational Reference2 : fl_lib/Mechanical/Translational Elements/Mechanical Translational Reference
  L : PMIOPort  Side=Right
  connections:
  Load Force/RConn1 -- Ideal Force Source/RConn1
  Mechanical Translational Reference2/LConn1 -- Ideal Force Source/RConn2
  Ideal Force Source/LConn1 -- L/RConn1

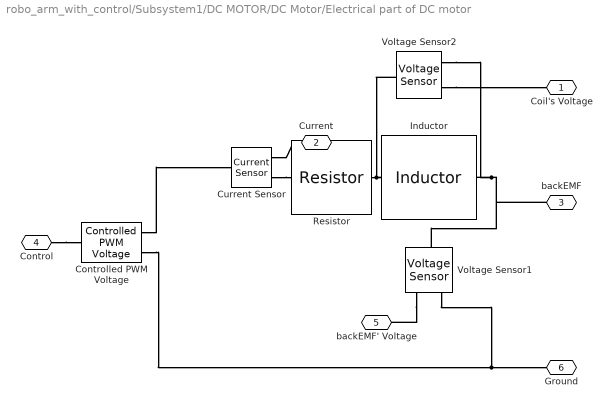
== system robo_arm_with_control/Subsystem1/DC MOTOR/DC Motor/Electrical part of DC motor ==
  Controlled PWM Voltage : elec_lib/Actuators & Drivers/Drivers/Controlled PWM Voltage  F=PWM_frequency Hz  TD=0 s  pulse_width_offset=0 s  pulse_min=0 s  Vmin=0 V  Vmax=5 V  Vm=PWM_amplitude V  pwm_or_av=1  event_type=1  sample_time=1e-6 s  u_min=0  u_max=1
      settings: SourceProductName=Simscape Electronics  SourceProductBaseCode=SN
  Current Sensor : fl_lib/Electrical/Electrical Sensors/Current Sensor
  Inductor : fl_lib/Electrical/Electrical Elements/Inductor  l=winding_inductance mH  r=0 Ohm  g=0 1/Ohm  i_specify=off  i_priority=None  i=0 A  i_nominal_specify=off  i_nominal_unit=A  i_nominal_value=1  v_specify=off  v_priority=None  v=0 V  v_nominal_specify=off  v_nominal_unit=V  v_nominal_value=1  i_L_specify=off  i_L_priority=High  i_L=0 A  i_L_nominal_specify=off  i_L_nominal_unit=A  i_L_nominal_value=1
  Resistor : fl_lib/Electrical/Electrical Elements/Resistor  R=winding_resistance Ohm  i_specify=off  i_priority=None  i=0 A  i_nominal_specify=off  i_nominal_unit=A  i_nominal_value=1  v_specify=off  v_priority=None  v=0 V  v_nominal_specify=off  v_nominal_unit=V  v_nominal_value=1
  Voltage Sensor1 : fl_lib/Electrical/Electrical Sensors/Voltage Sensor
  Voltage Sensor2 : fl_lib/Electrical/Electrical Sensors/Voltage Sensor
  Coil's Voltage : PMIOPort  Side=Right
  Current : PMIOPort  Port=2  Side=Right
  backEMF : PMIOPort  Port=3  Side=Left
  Control : PMIOPort  Port=4  Side=Right
  backEMF' Voltage : PMIOPort  Port=5  Side=Right
  Ground : PMIOPort  Port=6  Side=Right
  connections:
  Voltage Sensor2/RConn1 -- Coil's Voltage/RConn1
  Resistor/RConn1 -- Voltage Sensor2/LConn1 -- Inductor/LConn1
  Controlled PWM Voltage/RConn1 -- Current Sensor/LConn1
  Voltage Sensor1/RConn2 -- Controlled PWM Voltage/RConn2 -- Ground/RConn1
  Current Sensor/RConn1 -- Current/RConn1
  Voltage Sensor1/RConn1 -- backEMF' Voltage/RConn1
  Current Sensor/RConn2 -- Resistor/LConn1
  Voltage Sensor2/RConn2 -- Voltage Sensor1/LConn1 -- backEMF/RConn1 -- Inductor/RConn1
  Control/RConn1 -- Controlled PWM Voltage/LConn1

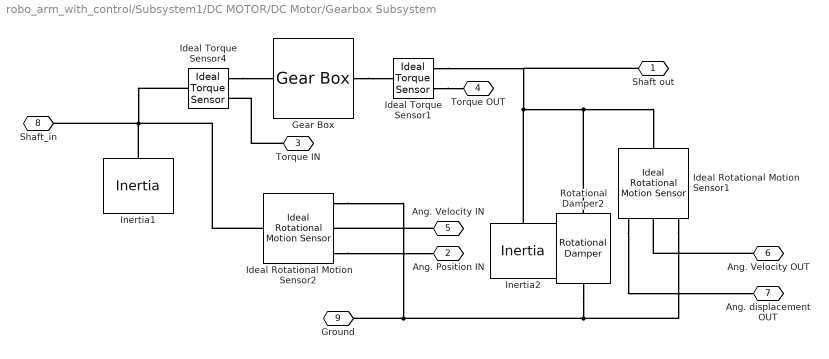
== system robo_arm_with_control/Subsystem1/DC MOTOR/DC Motor/Gearbox Subsystem ==
  Gear Box : fl_lib/Mechanical/Mechanisms/Gear Box  ratio=gear_ratio  t_in_specify=off  t_in_priority=None  t_in=0 N*m  t_in_nominal_specify=off  t_in_nominal_unit=N*m  t_in_nominal_value=1  t_out_specify=off  t_out_priority=None  t_out=0 N*m  t_out_nominal_specify=off  t_out_nominal_unit=N*m  t_out_nominal_value=1
  Ideal Rotational Motion Sensor1 : fl_lib/Mechanical/Mechanical Sensors/Ideal Rotational Motion Sensor  offset=0 rad
  Ideal Rotational Motion Sensor2 : fl_lib/Mechanical/Mechanical Sensors/Ideal Rotational Motion Sensor  offset=0 rad
  Ideal Torque Sensor1 : fl_lib/Mechanical/Mechanical Sensors/Ideal Torque Sensor
  Ideal Torque Sensor4 : fl_lib/Mechanical/Mechanical Sensors/Ideal Torque Sensor
  Inertia1 : fl_lib/Mechanical/Rotational Elements/Inertia  inertia=gear_1_inertia kg*m^2  w_specify=off  w_priority=High  w=0 rad/s  w_nominal_specify=off  w_nominal_unit=rad/s  w_nominal_value=1  t_specify=off  t_priority=None  t=0 N*m  t_nominal_specify=off  t_nominal_unit=N*m  t_nominal_value=1
  Inertia2 : fl_lib/Mechanical/Rotational Elements/Inertia  inertia=8000 g*cm^2  w_specify=off  w_priority=High  w=0 rad/s  w_nominal_specify=off  w_nominal_unit=rad/s  w_nominal_value=1  t_specify=off  t_priority=None  t=0 N*m  t_nominal_specify=off  t_nominal_unit=N*m  t_nominal_value=1
  Rotational Damper2 : fl_lib/Mechanical/Rotational Elements/Rotational Damper  D=gearbox_damping_factor N*m/(rad/s)  w_specify=off  w_priority=None  w=0 rad/s  w_nominal_specify=off  w_nominal_unit=rad/s  w_nominal_value=1  t_specify=off  t_priority=None  t=0 N*m  t_nominal_specify=off  t_nominal_unit=N*m  t_nominal_value=1
  Shaft out : PMIOPort  Side=Right
  Ang. Position IN : PMIOPort  Port=2  Side=Right
  Torque IN : PMIOPort  Port=3  Side=Right
  Torque OUT : PMIOPort  Port=4  Side=Right
  Ang. Velocity IN : PMIOPort  Port=5  Side=Right
  Ang. Velocity OUT : PMIOPort  Port=6  Side=Right
  Ang. displacement OUT : PMIOPort  Port=7  Side=Right
  Shaft_in : PMIOPort  Port=8  Side=Left
  Ground : PMIOPort  Port=9  Side=Left
  connections:
  Ang. Velocity IN/RConn1 -- Ideal Rotational Motion Sensor2/RConn2
  Inertia2/LConn1 -- Ideal Torque Sensor1/RConn1 -- Shaft out/RConn1 -- Rotational Damper2/LConn1 -- Ideal Rotational Motion Sensor1/LConn1
  Ideal Torque Sensor4/RConn1 -- Gear Box/LConn1
  Ideal Torque Sensor4/LConn1 -- Ideal Rotational Motion Sensor2/LConn1 -- Inertia1/LConn1 -- Shaft_in/RConn1
  Ideal Rotational Motion Sensor2/RConn3 -- Ang. Position IN/RConn1
  Ideal Torque Sensor1/RConn2 -- Torque OUT/RConn1
  Gear Box/RConn1 -- Ideal Torque Sensor1/LConn1
  Rotational Damper2/RConn1 -- Ideal Rotational Motion Sensor1/RConn1 -- Ideal Rotational Motion Sensor2/RConn1 -- Ground/RConn1
  Ideal Rotational Motion Sensor1/RConn3 -- Ang. displacement OUT/RConn1
  Torque IN/RConn1 -- Ideal Torque Sensor4/RConn2
  Ang. Velocity OUT/RConn1 -- Ideal Rotational Motion Sensor1/RConn2

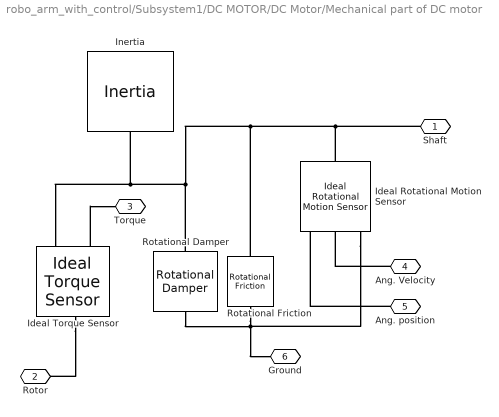
== system robo_arm_with_control/Subsystem1/DC MOTOR/DC Motor/Mechanical part of DC motor ==
  Ideal Rotational Motion Sensor : fl_lib/Mechanical/Mechanical Sensors/Ideal Rotational Motion Sensor  offset=0 rad
  Ideal Torque Sensor : fl_lib/Mechanical/Mechanical Sensors/Ideal Torque Sensor
  Inertia : fl_lib/Mechanical/Rotational Elements/Inertia  inertia=rotor_intertia kg*m^2  w_specify=off  w_priority=High  w=0 rad/s  w_nominal_specify=off  w_nominal_unit=rad/s  w_nominal_value=1  t_specify=off  t_priority=None  t=0 N*m  t_nominal_specify=off  t_nominal_unit=N*m  t_nominal_value=1
  Rotational Damper : fl_lib/Mechanical/Rotational Elements/Rotational Damper  D=0.00000954745 N*m/(rad/s)  w_specify=off  w_priority=None  w=0 rad/s  w_nominal_specify=off  w_nominal_unit=rad/s  w_nominal_value=1  t_specify=off  t_priority=None  t=0 N*m  t_nominal_specify=off  t_nominal_unit=N*m  t_nominal_value=1
  Rotational Friction : fl_lib/Mechanical/Rotational Elements/Rotational Friction  brkwy_trq=breakaway_friction_torque N*m  brkwy_vel=breakaway_friction_velocity rad/s  Col_trq=friction_torque N*m  visc_coef=0 N*m/(rad/s)  w_specify=off  w_priority=None  w=0 rad/s  w_nominal_specify=off  w_nominal_unit=rad/s  w_nominal_value=1  t_specify=off  t_priority=None  t=0 N*m  t_nominal_specify=off  t_nominal_unit=N*m  t_nominal_value=1
      settings: SourceProductName=Simscape
  Shaft : PMIOPort  Side=Right
  Rotor : PMIOPort  Port=2  Side=Left
  Torque : PMIOPort  Port=3  Side=Right
  Ang. Velocity : PMIOPort  Port=4  Side=Right
  Ang. position : PMIOPort  Port=5  Side=Right
  Ground : PMIOPort  Port=6  Side=Right
  connections:
  Ideal Torque Sensor/RConn2 -- Torque/RConn1
  Ideal Rotational Motion Sensor/RConn1 -- Ground/RConn1 -- Rotational Friction/RConn1 -- Rotational Damper/RConn1
  Ang. position/RConn1 -- Ideal Rotational Motion Sensor/RConn3
  Ideal Torque Sensor/LConn1 -- Rotor/RConn1
  Ideal Rotational Motion Sensor/LConn1 -- Rotational Damper/LConn1 -- Ideal Torque Sensor/RConn1 -- Inertia/LConn1 -- Rotational Friction/LConn1 -- Shaft/RConn1
  Ang. Velocity/RConn1 -- Ideal Rotational Motion Sensor/RConn2

== system robo_arm_with_control/Subsystem1/DC MOTOR/DC Motor/Subsystem ==
  torque_bf : Inport
  torque_af : Inport  Port=2
  speed_af : Inport  Port=3
  speed_af1 : Inport  Port=4
  Scope2 : Scope  NumInputPorts=4
  wires:
  torque_af/1 -> Scope2/2
  torque_bf/1 -> Scope2/1
  speed_af1/1 -> Scope2/4
  speed_af/1 -> Scope2/3

== system robo_arm_with_control/Subsystem1/Pneumatic Actuator/Double-Acting Actuator/Atm ==
  Temperature Source : fl_lib/Thermal/Thermal Sources/Temperature Source  temperature=T_atm K
      settings: SourceProductName=Simscape
  T : PMIOPort  Side=Right
  connections:
  Temperature Source/LConn1 -- T/RConn1

== system robo_arm_with_control/Subsystem1/Pneumatic Actuator/Double-Acting Actuator/Sensor ==
  Ideal Translational Motion Sensor : fl_lib/Mechanical/Mechanical Sensors/Ideal Translational Motion Sensor  offset=0 m
  Mechanical Translational Reference1 : fl_lib/Mechanical/Translational Elements/Mechanical Translational Reference
  PS-Simulink Converter : nesl_utility/PS-Simulink Converter  PhysicalDomain=network_engine_domain  SubClassName=ps_output  LeftPortType=input  RightPortType=output  PseudoPeriodic=off  Frequencies=[]  Unit=m  AffineConversion=off
  R : PMIOPort  Side=Left
  x : Outport
  wires:
  PS-Simulink Converter/1 -> x/1
  connections:
  Mechanical Translational Reference1/LConn1 -- Ideal Translational Motion Sensor/RConn1
  Ideal Translational Motion Sensor/LConn1 -- R/RConn1
  PS-Simulink Converter/LConn1 -- Ideal Translational Motion Sensor/RConn3

== stateflow chart robo_arm_with_control/Controller  ==
  settings: stateMachineType=MOORE_MACHINE
  state Start
    state Box_manipulation [parallel]
      settings: executionOrder=1
      state Pick_up_box
        state Arm_down
          Z_pos_out = 1;
        state Grab_box
          Z_pos_out = -1;
        (default) -> Start.Box_manipulation.Pick_up_box.Arm_down
        Start.Box_manipulation.Pick_up_box.Arm_down -> Start.Box_manipulation.Pick_up_box.Grab_box : [abs(z_sens - Z_pos_max) < 0.002]
      state Store_box
        box_waiting = 0;
        Y_pos_out = list_of_coordinates_y(mod(boxes_counter,n_cols)+1);
        X_pos_out = list_of_coordinates_x(floor(boxes_counter/n_cols)+1);
      state increment
        boxes_counter = boxes_counter+1
      state Go_to_start
        X_pos_out = 0;
        Y_pos_out = 0.45;
      state Drop_box
        state Arm_down
          Z_pos_out = 1;
        state Grab_box
          Z_pos_out = -1;
        (default) -> Start.Box_manipulation.Drop_box.Arm_down
        Start.Box_manipulation.Drop_box.Arm_down -> Start.Box_manipulation.Drop_box.Grab_box : [abs(z_sens - Z_pos_max) < 0.002]
      increment -> Pick_up_box
      Start.Box_manipulation.Pick_up_box.Grab_box -> Store_box : [abs(Z_pos_min - z_sens) < 0.002]
      (default) -> Go_to_start
      Go_to_start -> increment : [abs(x_sens - X_pos_out) < 0.01 && abs(y_sens -Y_pos_out) < 0.01 && box_waiting==1]
      Store_box -> Drop_box : [abs(y_sens -Y_pos_out) < 0.01 && abs(x_sens -X_pos_out) < 0.01]
      Start.Box_manipulation.Drop_box.Grab_box -> Go_to_start : [abs(z_sens - Z_pos_min) < 0.002]
    state Box_arrived [parallel]
      if boxes_counter ~= n_cols*n_rows
      box_waiting=1;
      end
      settings: executionOrder=2
  (default) -> Start
  data: x_sens input; Y_pos_out output =0; y_sens input; Z_pos_max constant double =0.4; X_pos_out output =-0.5; z_sens input; Z_pos_out output =0; Z_pos_min constant double =0; box_arrived input; n_cols constant double =n_cols; n_rows constant double =n_rows; box_waiting local; list_of_coordinates_x constant double size=n_rows =list_of_coordinates_x; list_of_coordinates_y constant double size=n_cols =list_of_coordinates_y; boxes_counter local =0
